simulink model "qpsk"  (R2022b)
settings: Solver=ode45  StartTime=0.0  StopTime=10  FixedStep=1/64000/20  RelTol=1e-3  EnableMultiTasking=on
undefined symbols (not defined in the file or in its folder): gcbh, rcfiltgaincompat
libraries: commfilt2 x2, dspsigops x2, commchan3 x1, commsink2 x1, dspindex x1, commrandsrc2 x1
settings Model: Creator=ssd  LastModifiedBy=水月镜花
settings SolverCC: AlgebraicLoopSolver=TrustRegion
settings DataIOCC: LimitDataPoints=on  SaveFormat=Array  SignalLoggingSaveFormat=ModelDataLogs  ReturnWorkspaceOutputs=off
settings OptimizationCC: ExpressionDepthLimit=2147483647  InitFltsAndDblsToZero=on  LifeSpan=inf
settings DebuggingCC: UnderspecifiedInitializationDetection=Classic  MergeDetectMultiDrivingBlocksExec=none  SolverPrmCheckMsg=warning  FcnCallInpInsideContextMsg=warning  UnconnectedInputMsg=warning  UnconnectedOutputMsg=warning  UnconnectedLineMsg=warning  StateNameClashWarn=warning  SFUnexpectedBacktrackingDiag=warning  SFNoUnconditionalDefaultTransitionDiag=warning  SFExecutionAtInitializationDiag=none  SFMachineParentedDataDiag=warning  ArithmeticOperatorsInVariantConditions=warning
settings HardwareCC: ProdBitPerPointer=32  ProdBitPerSizeT=32  ProdBitPerPtrDiffT=32  ProdLargestAtomicFloat=None  ProdIntDivRoundTo=Undefined  ProdEndianess=Unspecified  ProdWordSize=32  ProdHWDeviceType=32-bit Generic
settings ModelReferenceCC: EnableRefExpFcnMdlSchedulingChecks=on  PropagateSignalLabelsOutOfModel=off
settings SFSimCC: SimUseLocalCustomCode=off  SimParseCustomCode=off  CustomCodeUndefinedFunction=UseInterfaceOnly
settings RTWCC: RTWUseLocalCustomCode=off
settings CodeAppCC: StateflowObjectComments=on
settings GRTTargetCC: TargetLangStandard=C89/C90 (ANSI)  CombineOutputUpdateFcns=off  GRTInterface=on
settings ConfigComp: CovMetricSettings=dw  CovSaveCumulativeToWorkspaceVar=on  CovSaveSingleToWorkspaceVar=on  CovExternalEMLEnable=off

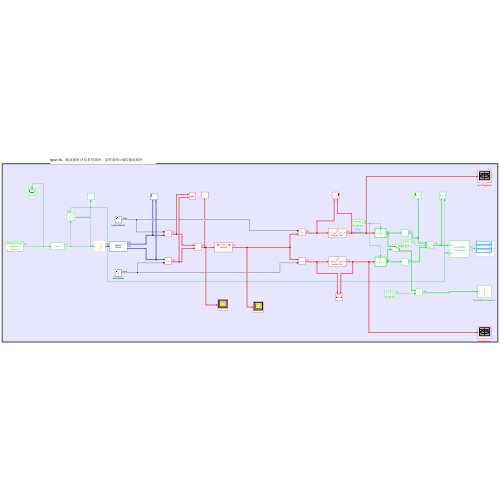
[thumbnail: Simulink's stored preview of the top-level diagram]
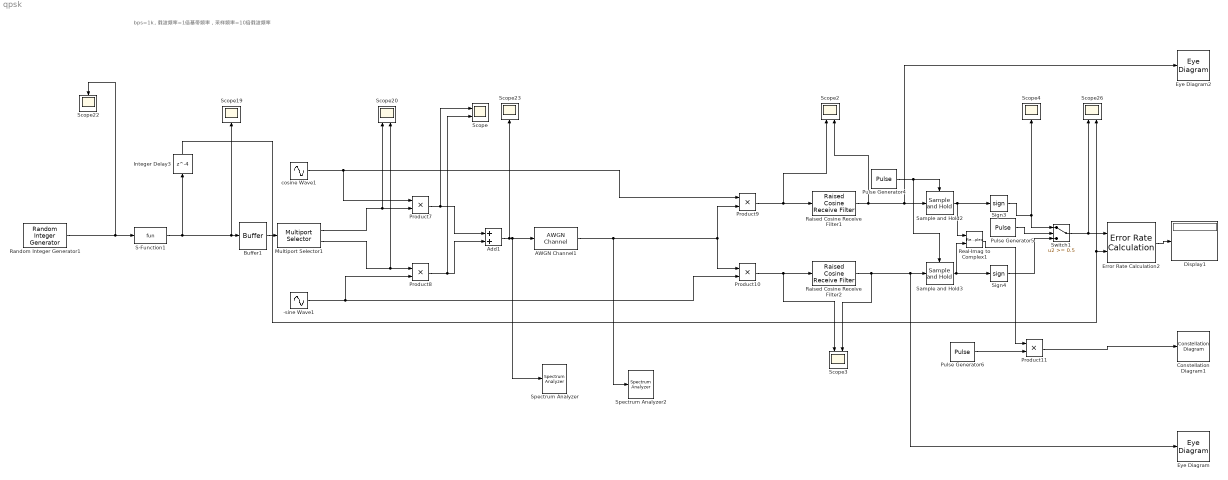
== system qpsk ==
  note: bps=1k，载波频率=1倍基带频率，采样频率=10倍载波频率
  -sine Wave1 : Sin  Frequency=2*pi*1000  Phase=pi  SampleTime=0
  AWGN Channel1 : commchan3/AWGN Channel  InputProcessing=Columns as channels (frame based)  seed=67  noiseMode="Signal to noise ratio  (SNR)"  EbNodB=EbNo  EsNodB=0  SNRdB=30  bitsPerSym=2  Ps=1  Tsym=0.002  variance=1
  Add1 : Sum  SampleTime=1/10000
  Buffer1 : Buffer  N=2
  Constellation Diagram1 : ConstellationDiagram  WindowPosition=[641.000000,292.000000,591.000000,544.000000,]  ScopeFrameLocation=window  SymbolsToDisplaySource=Property  SymbolsToDisplay=10000  ReferenceConstellation=QPSK  XLimits=[-2.618432219563941,3.4872027474968688]  YLimits=[-2.618432219563941,3.4872027474968688]  DefaultConfigurationName=comm.scopes.ConstellationDiagramBlockCfg
  Display1 : Display
      settings: SampleTime=0.1
  Error Rate Calculation2 : commsink2/Error Rate Calculation  N=0  st_delay=0  cp_mode=Entire frame  subframe=[]  PMode=Port  WsName=ErrorVec  RsMode2=off  stop=off  numErr=100  maxBits=1e6
  Eye Diagram : EyeDiagram
  Eye Diagram2 : EyeDiagram
  Integer Delay3 : Delay  DelayLength=4  SampleTime=1/1000
  Multiport Selector1 : dspindex/Multiport Selector  rowsOrCols=Rows  idxCellArray={1 2}  idxErrMode=Clip Index
  Product{7..10} (4 alike) : Product  RndMeth=Zero  SampleTime=1/10000
  Product11 : Product  RndMeth=Zero  SampleTime=1/1000
  Pulse Generator4 : DiscretePulseGenerator  SampleTime=1/1000
  Pulse Generator5 : DiscretePulseGenerator  SampleTime=1/1000
  Pulse Generator6 : DiscretePulseGenerator  Amplitude=0.45  SampleTime=1/1000
  Raised Cosine Receive Filter1 : commfilt2/Raised Cosine Receive Filter  filtType=Square root  R=0.5  filtSpan=2*(2)  N=10  downFactor=1  downOffset=0  filterGain=(1.5)*rcfiltgaincompat(gcbh)  InputProcessing=Columns as channels (frame based)  RateOptions=Allow multirate processing  framing=Mute  checkCoeff=off  variableName=rcRxFilt1  currentFiltSpan=2*(2)  D=2  inputOffset=0  sampMode=Mute  saveAsFlag=0  rateMode=Downsampling  checkGain=User-specified  launchFVT=off  roundingMode=Floor  overflowMode=off  coeffDataTypeStr=Inherit: Same word length as input  coeffMin=[]  coeffMax=[]  coeffLastDataTypeStr=Inherit: Same word length as input  accumDataTypeStr=Inherit: Same as product output  accumLastDataTypeStr=Inherit: Same as product output  outputDataTypeStr=Inherit: Same as accumulator  outputMin=[]  outputMax=[]  outputLastDataTypeStr=Inherit: Same as accumulator
      link override Check Signal Attributes: Frame=Sample-based  Dimensions=Scalar (1-D or 2-D)
      link override Downsample: smode=Allow multirate  fmode=Maintain input frame size
  Raised Cosine Receive Filter2 : commfilt2/Raised Cosine Receive Filter  filtType=Square root  R=0.5  filtSpan=2*(2)  N=10  downFactor=1  downOffset=0  filterGain=(1.5)*rcfiltgaincompat(gcbh)  InputProcessing=Columns as channels (frame based)  RateOptions=Allow multirate processing  framing=Mute  checkCoeff=off  variableName=rcRxFilt2  currentFiltSpan=2*(2)  D=2  inputOffset=0  sampMode=Mute  saveAsFlag=0  rateMode=Downsampling  checkGain=User-specified  launchFVT=off  roundingMode=Floor  overflowMode=off  coeffDataTypeStr=Inherit: Same word length as input  coeffMin=[]  coeffMax=[]  coeffLastDataTypeStr=Inherit: Same word length as input  accumDataTypeStr=Inherit: Same as product output  accumLastDataTypeStr=Inherit: Same as product output  outputDataTypeStr=Inherit: Same as accumulator  outputMin=[]  outputMax=[]  outputLastDataTypeStr=Inherit: Same as accumulator
      link override Check Signal Attributes: Frame=Sample-based  Dimensions=Scalar (1-D or 2-D)
      link override Downsample: smode=Allow multirate  fmode=Maintain input frame size
  Random Integer Generator1 : commrandsrc2/Random Integer Generator  mul=2  seed=37  Ts=1/1000  frameBased=off  sampPerFrame=1  orient=off  outDataType=double
  Real-Imag to Complex1 : RealImagToComplex
  S-Function1 : S-Function  FunctionName=fun  SFunctionDeploymentMode=off  EnableBusSupport=off
  Sample and Hold2 : dspsigops/Sample and Hold  trig=Rising edge  initCond=0  latchinput=off
  Sample and Hold3 : dspsigops/Sample and Hold  trig=Rising edge  initCond=0  latchinput=off
  Scope{,2..3,20,26} (5 alike) : Scope  NumInputPorts=2
  Scope{4,19,22..23} (4 alike) : Scope
  Sign3 : Signum
  Sign4 : Signum
  Spectrum Analyzer : SpectrumAnalyzer
  Spectrum Analyzer2 : SpectrumAnalyzer
  Switch1 : Switch  Threshold=0.5  SaturateOnIntegerOverflow=off  InputSameDT=off
  cosine Wave1 : Sin  Frequency=2*pi*1000  Phase=pi/2  SampleTime=0
  wires:
  Random Integer Generator1/1 -> S-Function1/1, Scope22/1
  Buffer1/1 -> Multiport Selector1/1
  S-Function1/1 -> Scope19/1, Buffer1/1, Integer Delay3/1
  Multiport Selector1/1 -> Scope20/1, Product7/2
  Multiport Selector1/2 -> Scope20/2, Product8/1
  Product7/1 -> Scope/1, Add1/1
  Product8/1 -> Scope/2, Add1/2
  Add1/1 -> Spectrum Analyzer/1, AWGN Channel1/1, Scope23/1
  AWGN Channel1/1 -> Product10/1, Product9/2, Spectrum Analyzer2/1
  -sine Wave1/1 -> Product8/2, Product10/2
  Product9/1 -> Scope2/1, Raised Cosine Receive Filter1/1
  Product10/1 -> Raised Cosine Receive Filter2/1, Scope3/1
  Raised Cosine Receive Filter1/1 -> Eye Diagram2/1, Sample and Hold2/1, Scope2/2
  Pulse Generator4/1 -> Sample and Hold3/Trigger, Sample and Hold2/Trigger
  Sample and Hold2/1 -> Real-Imag to Complex1/1, Sign3/1
  Sample and Hold3/1 -> Sign4/1, Real-Imag to Complex1/2
  Sign3/1 -> Switch1/1, Scope4/1
  Sign4/1 -> Switch1/3
  Pulse Generator5/1 -> Switch1/2
  Switch1/1 -> Error Rate Calculation2/1, Scope26/1
  Real-Imag to Complex1/1 -> Product11/1
  Pulse Generator6/1 -> Product11/2
  Product11/1 -> Constellation Diagram1/1
  Error Rate Calculation2/1 -> Display1/1
  Raised Cosine Receive Filter2/1 -> Eye Diagram/1, Sample and Hold3/1, Scope3/2
  cosine Wave1/1 -> Product9/1, Product7/1
  Integer Delay3/1 -> Error Rate Calculation2/2, Scope26/2
